simulink model "modulation_example_qam_bpsk"  (R2015b)
settings: Solver=VariableStepAuto  StartTime=0.0  StopTime=0.01  RelTol=1e-3
undefined symbols (not defined in the file or in its folder): i
libraries: commanapbnd3 x3, commdigbbndpm3 x2, commdigbbndam3 x2, commseqgen3 x1, commrandsrc3 x1
settings Model: Creator=liujj-d  LastModifiedBy=liujj-d

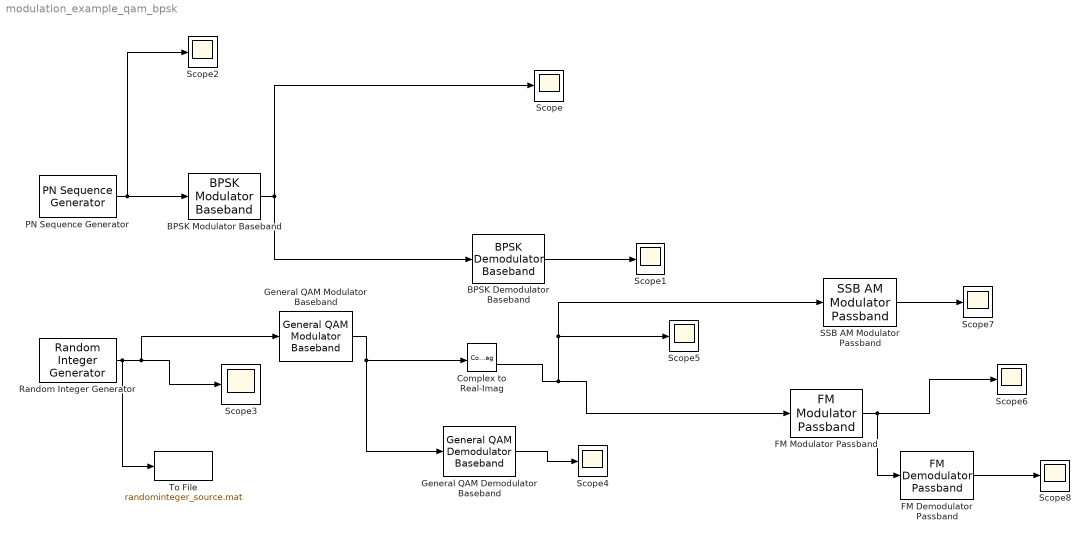
== system modulation_example_qam_bpsk ==
  BPSK Demodulator Baseband : commdigbbndpm3/BPSK Demodulator Baseband  Ph=0  DecType=Hard decision  VarSource=Dialog  Variance=1  outDtype=Inherit via internal rule  derotateFactorWordLen=16
  BPSK Modulator Baseband : commdigbbndpm3/BPSK Modulator Baseband  Ph=0  outDtype=double  outWordLen=16  outUDDataType=sfix(16)  outFracLenMode=Best precision  outFracLen=15
  Complex to Real-Imag : ComplexToRealImag
  FM Demodulator Passband : commanapbnd3/FM Demodulator Passband  Fc=100  Ph=0  Kc=30  Ho=10
  FM Modulator Passband : commanapbnd3/FM Modulator Passband  Fc=100  Ph=0  Kc=100
  General QAM Demodulator Baseband : commdigbbndam3/General QAM Demodulator Baseband  SigCon=[exp(2*pi*i*[0:15]/16)]  OutType=Integer  DecType=Hard decision  VarSource=Dialog  Variance=1  outDtypeBit=Inherit via internal rule  outDtype=Inherit via internal rule  roundingMode=Floor  overflowMode=Wrap  sigConstWordLen=16  accum1WordLen=32  accum1FracLen=30  prodInWordLen=32  prodInFracLen=30  prodOutWordLen=32  prodOutFracLen=30  accum2WordLen=32  accum2FracLen=30  accum3WordLen=32  accum3FracLen=30  nsiWordLen=32  nsiFracLen=30  invn0WordLen=16  invn0FracLen=8  outputWordLen=32  outputFracLen=30
  General QAM Modulator Baseband : commdigbbndam3/General QAM Modulator Baseband  SigCon=[exp(2*pi*i*[0:15]/16)]  outDtype=double  outWordLen=16  outUDDataType=sfix(16)  outFracLenMode=Best precision  outFracLen=15
  PN Sequence Generator : commseqgen3/PN Sequence Generator  poly='z^6 + z + 1'  ini_sta=[0 0 0 0 0 1]  outBitMaskSource=Dialog parameter  shift=0  outVarSiz=off  maxOutSizeMode=Dialog parameter  maxOutSize=[10 1]  Ts=1  sampPerFrame=1  reset=off  bitPackedOutputs=off  outDataType=double  numPackedBits=8  bitPackDataSigned=off  bitPackedOutDType=double
  Random Integer Generator : commrandsrc3/Random Integer Generator  SetSize=16  SeedSource=Auto  Seed=0  SampleTime=.0001  SamplesPerFrame=1  OutputDataType=uint8  SimulateUsing=Interpreted execution
  SSB AM Modulator Passband : commanapbnd3/SSB AM Modulator Passband  Fc=300  Ph=0  Sd=Upper  Ho=100
  Scope{,1..8} (9 alike) : Scope
  To File : ToFile  Filename=randominteger_source.mat  MatrixName=randint  SaveFormat=Timeseries
      settings: Decimation=1000
  wires:
  PN Sequence Generator/1 -> Scope2/1, BPSK Modulator Baseband/1
  BPSK Modulator Baseband/1 -> BPSK Demodulator Baseband/1, Scope/1
  BPSK Demodulator Baseband/1 -> Scope1/1
  General QAM Modulator Baseband/1 -> Complex to Real-Imag/1, General QAM Demodulator Baseband/1
  General QAM Demodulator Baseband/1 -> Scope4/1
  Random Integer Generator/1 -> To File/1, General QAM Modulator Baseband/1, Scope3/1
  SSB AM Modulator Passband/1 -> Scope7/1
  FM Modulator Passband/1 -> FM Demodulator Passband/1, Scope6/1
  Complex to Real-Imag/2 -> Scope5/1, SSB AM Modulator Passband/1, FM Modulator Passband/1
  FM Demodulator Passband/1 -> Scope8/1
